simulink model "Neural network based MRAC"  (R2015b)
settings: Solver=ode45  StartTime=0.0  StopTime=50  RelTol=1e-3
settings Model: Creator=Administrator  LastModifiedBy=Akhil Jarodia
settings DataIOCC: SaveFormat=Array
settings DebuggingCC: SolverPrmCheckMsg=warning
settings HardwareCC: ProdBitPerPointer=32  ProdLargestAtomicFloat=None  ProdIntDivRoundTo=Undefined  ProdEndianess=Unspecified  ProdWordSize=32  ProdHWDeviceType=32-bit Generic
settings GRTTargetCC: GeneratePreprocessorConditionals=Disable all
settings ConfigComp: CovModelRefEnable=Off  CovSFcnEnable=off

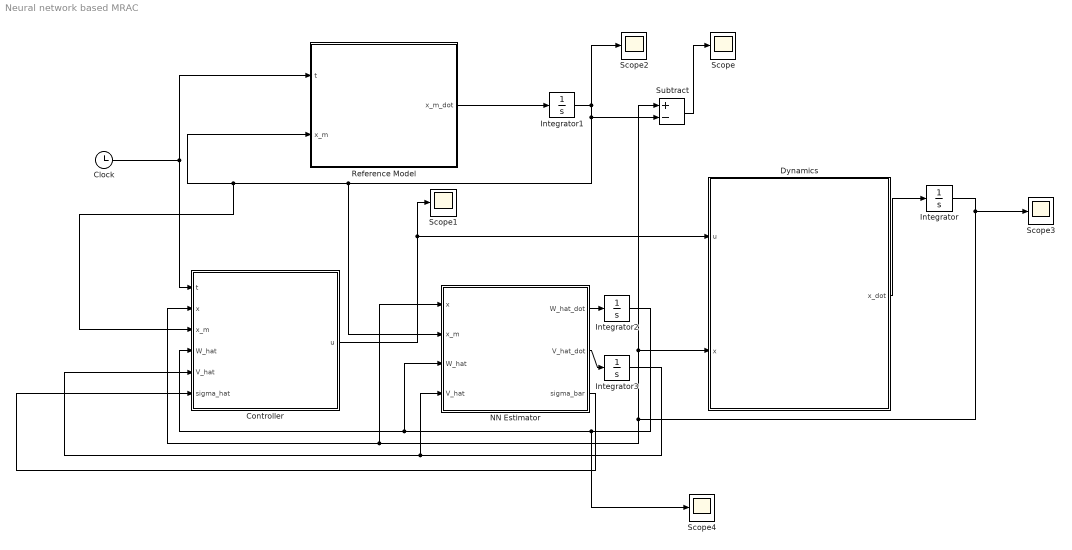
== system Neural network based MRAC ==
  Clock : Clock
      settings: Decimation=50
  Controller : MATLAB Function  TreatAsAtomicUnit=on
  Dynamics : MATLAB Function  TreatAsAtomicUnit=on
  Integrator : Integrator  InitialCondition=[-1;1]
  Integrator1 : Integrator  InitialCondition=[0;0]
  Integrator2 : Integrator  InitialCondition=zeros(11,1)
  Integrator3 : Integrator  InitialCondition=zeros(3,10)
  NN Estimator : MATLAB Function  TreatAsAtomicUnit=on
  Reference Model : MATLAB Function  TreatAsAtomicUnit=on
  Scope{,1..4} (5 alike) : Scope
  Subtract : Sum  Inputs=+-
  wires:
  Dynamics/1(x_dot) -> Integrator/1
  Integrator/1 -> Scope3/1, Subtract/1, Dynamics/2(x), NN Estimator/1(x), Controller/2(x)
  Clock/1 -> Controller/1(t), Reference Model/1(t)
  Controller/1(u) -> Scope1/1, Dynamics/1(u)
  Reference Model/1(x_m_dot) -> Integrator1/1
  NN Estimator/1(W_hat_dot) -> Integrator2/1
  Integrator2/1 -> Scope4/1, NN Estimator/3(W_hat), Controller/4(W_hat)
  Subtract/1 -> Scope/1
  NN Estimator/2(V_hat_dot) -> Integrator3/1
  Integrator3/1 -> NN Estimator/4(V_hat), Controller/5(V_hat)
  Integrator1/1 -> Scope2/1, NN Estimator/2(x_m), Controller/3(x_m), Reference Model/2(x_m), Subtract/2
  NN Estimator/3(sigma_bar) -> Controller/6(sigma_hat)

== matlab function Neural network based MRAC/Controller ==
  data: u output; t input; x input; x_m input; W_hat input; V_hat input; sigma_hat input
function u  = controller(t,x,x_m,W_hat, V_hat,sigma_hat)

e=x-x_m;
%r=10;
%r=exp(-t);
r=sin(t);
%r=2*sin(t);
k_s=2;
k_x=[-2/3 -1/3]'; % note that the linear control gain is directly chosen instead of adapting with an assumption of $A$ matrix to be known
L_delta_a=3;
B=[0;L_delta_a];
P=[3.5 0.5; 0.5 1.5];
delta_hat=W_hat' * sigma_hat;
% u=k_x'*x+r-W_hat'*V_hat;
u=k_x'*x + r - delta_hat- k_s*B'*P*e;
end

== matlab function Neural network based MRAC/Dynamics ==
  data: u input; x input; x_dot output
function x_dot   = dynamics(u,x)
%#codegen
L_delta_a=3;
A=[0 1; 0 0];
B=[0;L_delta_a];
a0=0.8;
a1=0.2314;
a2=0.6918;
a3=-0.6245;
a4=0.0095;
a5=0.0214;

theta=x(1,1);
p=x(2,1);

delta=a0+a1*theta+a2*p+a3*abs(theta)*p+a4*abs(p)*p+a5*theta^3;
x_dot=A*x+B*(u+delta/L_delta_a);
end

== matlab function Neural network based MRAC/NN Estimator ==
  data: W_hat_dot output; x input; x_m input; V_hat_dot output; W_hat input; V_hat input; sigma_bar output
function [W_hat_dot, V_hat_dot,sigma_bar]   = NN_estimator(x,x_m,W_hat,V_hat)

e=x-x_m; % tracking error 
L=10; % number of neurons
gamma_w=eye(L+1);
gamma_v=eye(3);
sigma_w=2;
sigma_v=2;


P=[3.5 0.5; 0.5 1.5]; % the command P=lyap(A_m',Q) is used to calculate P. In this case Q is chosen as Q=2*eye(2). 
L_delta_a=3;
B=[0;L_delta_a];
sigma=(1/(1+exp(-1*(V_hat' * [1;x]))));
sigma_bar=[1 sigma]';
sigma_bar_hat_dot=diag(sigma.*(1-sigma));
sigma_bar_hat_dot=[zeros(1,size(sigma_bar_hat_dot,2));sigma_bar_hat_dot];

v2=sigma_bar_hat_dot*V_hat'*[1;x];
W_hat_dot=(gamma_w*(sigma_bar-v2)* e' * P* B ) - gamma_w*sigma_w*W_hat;
V_hat_dot=(gamma_v * [1;x]* e' * P * B* W_hat' * sigma_bar_hat_dot) - (gamma_v * sigma_v * V_hat);

== matlab function Neural network based MRAC/Reference Model ==
  data: x_m_dot output; t input; x_m input
function x_m_dot  = reference(t,x_m)
am1=-2;
am2=-1;
L_delta_a=3;
%r=exp(-t);
r=sin(t);
%r=2*sin(t);
A_m=[0 1; am1 am2];
B_m=[0; L_delta_a];
x_m_dot=A_m*x_m+B_m*r;
